simulink subsystem "suspensionTwoDOFLateral"  (R2023a)
settings: Solver=VariableStepAuto  StartTime=0.0  StopTime=10.0  RelTol=1e-3
model mask{obj=obj}
  mask prompts: obj "Spring Object:"
settings Model: Creator=grouleau  LastModifiedBy=grouleau

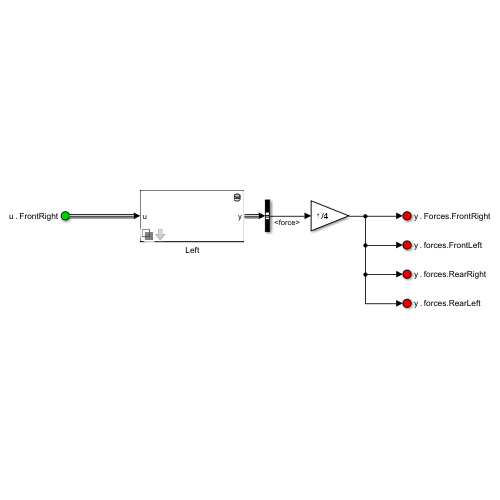
[thumbnail: Simulink's stored preview of the top-level diagram]
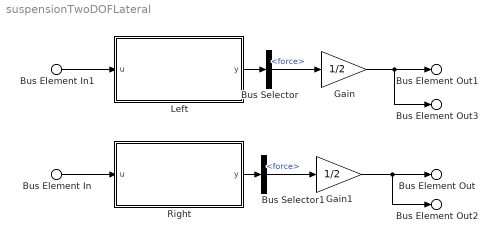
== system suspensionTwoDOFLateral ==
  Bus Element In : Inport  PortName=u  Element=FrontRight
  Bus Element In1 : Inport  PortName=u  Element=FrontLeft
  Bus Selector : BusSelector  OutputSignals=force
  Bus Selector1 : BusSelector  OutputSignals=force
  Gain : Gain  Gain=1/2
  Gain1 : Gain  Gain=1/2
  Left : Subsystem  Variant=on  VariantChoicesSpecifier=obj.getVariantChoices()  VariantControlMode=label  LabelModeActiveChoice=suspension  mask{obj=obj.Left}
      mask prompts: obj "Part Object"
  Right : Subsystem  Variant=on  VariantChoicesSpecifier=obj.getVariantChoices()  VariantControlMode=label  LabelModeActiveChoice=suspension  mask{obj=obj.Right}
      mask prompts: obj "Part Object"
  Bus Element Out1 : Outport  PortName=y  Element=Forces.FrontLeft
  Bus Element Out3 : Outport  PortName=y  Element=Forces.RearLeft
  Bus Element Out : Outport  PortName=y  Element=Forces.FrontRight
  Bus Element Out2 : Outport  PortName=y  Element=Forces.RearRight
  wires:
  Bus Selector/1 -> Gain/1  "<force>"
  Left/1(y) -> Bus Selector/1
  Bus Element In/1 -> Right/1(u)
  Bus Element In1/1 -> Left/1(u)
  Bus Selector1/1 -> Gain1/1  "<force>"
  Right/1(y) -> Bus Selector1/1
  Gain/1 -> Bus Element Out1/1, Bus Element Out3/1
  Gain1/1 -> Bus Element Out2/1, Bus Element Out/1

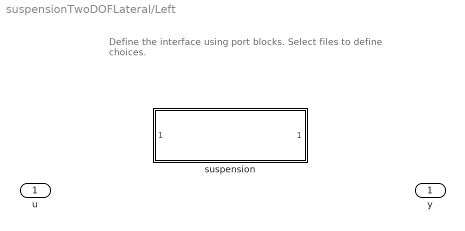
== system suspensionTwoDOFLateral/Left ==
  note: Define the interface using port blocks.
      | Select files to define choices.
  u : Inport
  suspension : Subsystem  VariantControl=suspension  ReferencedSubsystem=suspension  obj=obj
  y : Outport

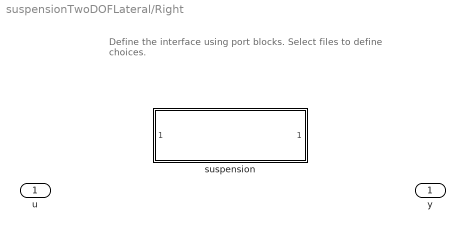
== system suspensionTwoDOFLateral/Right ==
  note: Define the interface using port blocks.
      | Select files to define choices.
  u : Inport
  suspension : Subsystem  VariantControl=suspension  ReferencedSubsystem=suspension  obj=obj
  y : Outport
